simulink model "SubSistemaTermico"  (R2023b)
settings: Solver=VariableStepAuto  StartTime=0.0  StopTime=10.0  RelTol=1e-3
values from neighbouring files (symbols this model uses):
  alpha_cu = 3.9e-3    (= 0.0039)    [parametros_proyecto2.m]
  Cts = 0.818    [parametros_proyecto2.m]
  Rs_ref = 1.02    [parametros_proyecto2.m]
  Rts_amb = 146.7    [parametros_proyecto2.m]
  Ts0 = 25    [parametros_proyecto2.m]
undefined symbols (not defined in the file or in its folder): magnitude
settings Model: Creator=ignab  LastModifiedBy=ignab

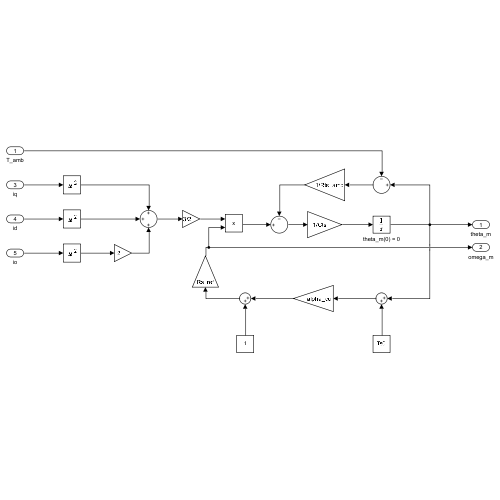
[thumbnail: Simulink's stored preview of the top-level diagram]
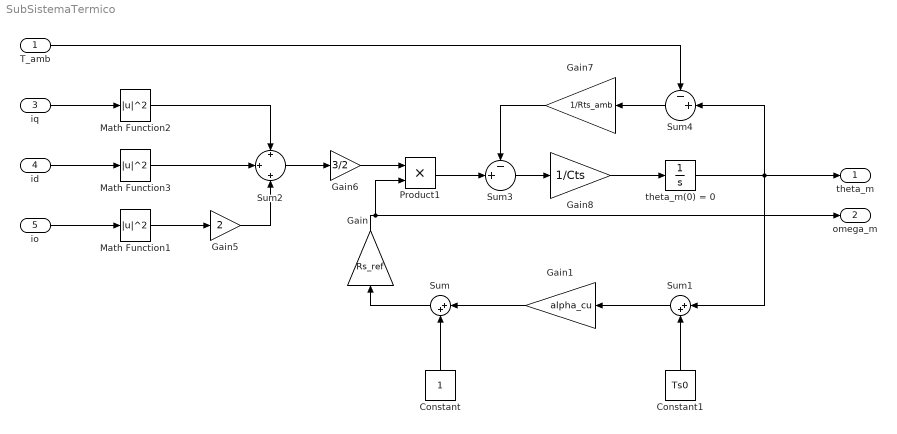
== system SubSistemaTermico ==
  T_amb : Inport
  iq : Inport  Port=3
  id : Inport  Port=4
  io : Inport  Port=5
  Constant : Constant
  Constant1 : Constant  Value=Ts0
  Gain : Gain  Gain=Rs_ref
  Gain1 : Gain  Gain=alpha_cu
  Gain5 : Gain  Gain=2
  Gain6 : Gain  Gain=3/2
  Gain7 : Gain  Gain=1/Rts_amb
  Gain8 : Gain  Gain=1/Cts
  Math Function1 : Math  Operator=magnitude^2  OutputSignalType=real
  Math Function2 : Math  Operator=magnitude^2  OutputSignalType=real
  Math Function3 : Math  Operator=magnitude^2  OutputSignalType=real
  Product1 : Product
  Sum : Sum  Inputs=|++
  Sum1 : Sum  Inputs=|++
  Sum2 : Sum  Inputs=+|+|+
  Sum3 : Sum  Inputs=-+|
  Sum4 : Sum  Inputs=-+|
  theta_m(0) = 0 : Integrator
  theta_m : Outport
  omega_m : Outport  Port=2
  wires:
  Gain5/1 -> Sum2/3
  Math Function3/1 -> Sum2/2
  Math Function2/1 -> Sum2/1
  Math Function1/1 -> Gain5/1
  Sum2/1 -> Gain6/1
  Gain6/1 -> Product1/1
  Gain/1 -> omega_m/1, Product1/2
  Gain1/1 -> Sum/1
  Sum1/1 -> Gain1/1
  Constant/1 -> Sum/2
  Constant1/1 -> Sum1/2
  Sum/1 -> Gain/1
  Sum3/1 -> Gain8/1
  Product1/1 -> Sum3/2
  Gain8/1 -> theta_m(0) = 0/1
  theta_m(0) = 0/1 -> Sum4/2, Sum1/1, theta_m/1
  Gain7/1 -> Sum3/1
  Sum4/1 -> Gain7/1
  T_amb/1 -> Sum4/1
  iq/1 -> Math Function2/1
  id/1 -> Math Function3/1
  io/1 -> Math Function1/1
